simulink model "FM_Modulation_Sim (3)"  (R2023b)
settings: Solver=FixedStepAuto  StartTime=0.0  StopTime=0.003  FixedStep=0.000001  RelTol=1e-3
settings Model: Creator=mahil  LastModifiedBy=ASUS

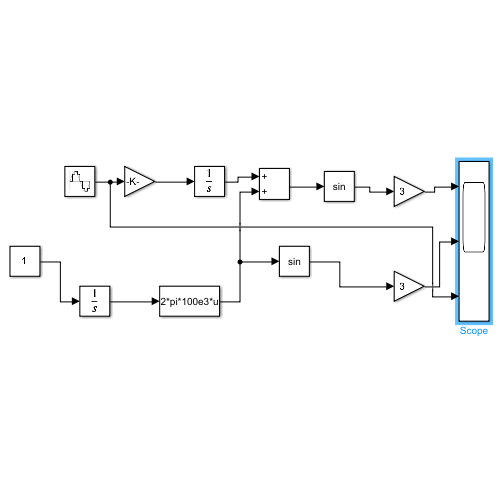
[thumbnail: Simulink's stored preview of the top-level diagram]
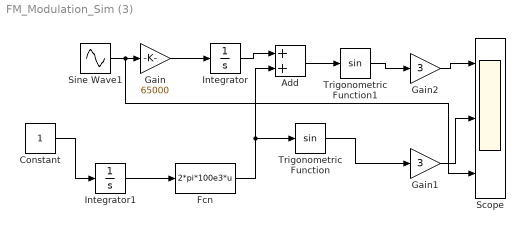
== system FM_Modulation_Sim (3) ==
  Add : Sum
  Constant : Constant
  Fcn : Fcn  Expr=2*pi*100e3*u
  Gain : Gain  Gain=65000
  Gain1 : Gain  Gain=3
  Gain2 : Gain  Gain=3
  Integrator : Integrator
  Integrator1 : Integrator
  Scope : Scope  NumInputPorts=3
  Sine Wave1 : Sin  Amplitude=3  Frequency=2*pi*4000  SampleTime=0.000001
  Trigonometric Function : Trigonometry
  Trigonometric Function1 : Trigonometry
  wires:
  Trigonometric Function/1 -> Gain1/1
  Trigonometric Function1/1 -> Gain2/1
  Add/1 -> Trigonometric Function1/1
  Integrator/1 -> Add/1
  Fcn/1 -> Trigonometric Function/1, Add/2
  Integrator1/1 -> Fcn/1
  Constant/1 -> Integrator1/1
  Sine Wave1/1 -> Scope/3, Gain/1
  Gain/1 -> Integrator/1
  Gain2/1 -> Scope/1
  Gain1/1 -> Scope/2
